simulink model "HoodReleaseModel"  (R2020b)
settings: Solver=VariableStepAuto  StartTime=0.0  StopTime=inf  RelTol=1e-3
libraries: simulink x2
settings Model: Creator=99003785  LastModifiedBy=99003785

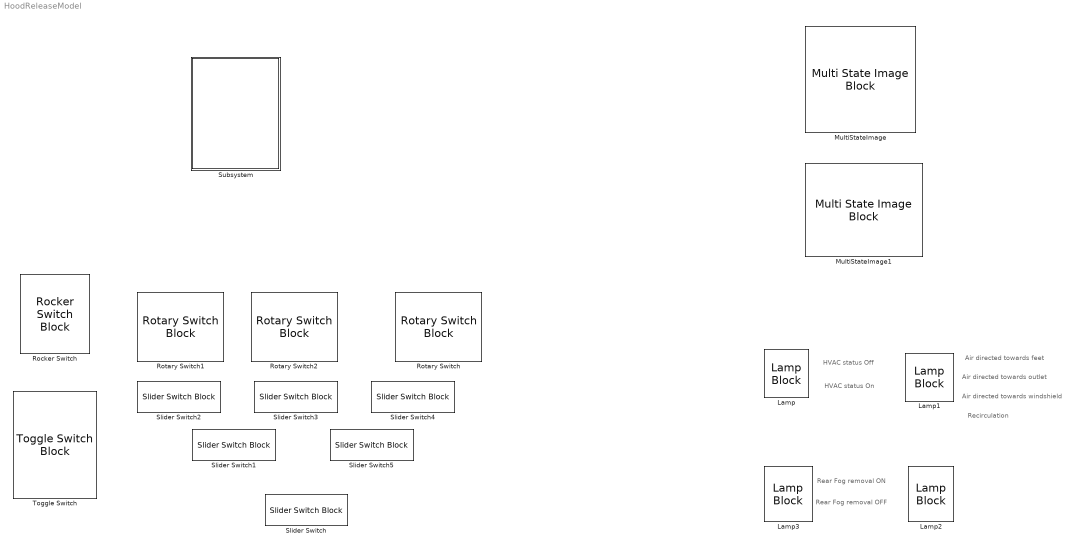
== system HoodReleaseModel ==
  note: Rear Fog removal OFF
  note: Rear Fog removal ON
  note: Recirculation
  note: Air directed towards windshield
  note: Air directed towards outlet
  note: Air directed towards feet
  note: HVAC status Off
  note: HVAC status On
  Lamp{,1..3} (4 alike) : LampBlock
  MultiStateImage : MultiStateImageBlock
  MultiStateImage1 : MultiStateImageBlock
  Rocker Switch : RockerSwitchBlock
      settings: Values={{'On', 'Off'}, [1 0]}
  Rotary Switch : RotarySwitchBlock
      settings: Values={{'Off', 'Low', 'Medium', 'High'}, [0 1 2 3]}
  Rotary Switch1 : RotarySwitchBlock
      settings: Values={{'Off', 'Low', 'Medium', 'High'}, [0 1 2 3]}
  Rotary Switch2 : RotarySwitchBlock
      settings: Values={{'Off', 'AC', 'Heater', 'Air-Vent'}, [0 1 2 3]}
  Slider Switch{,1..5} (6 alike) : SliderSwitchBlock
      settings: Values={{'Off', 'On'}, [0 1]}
  Subsystem : Subsystem
  Toggle Switch : ToggleSwitchBlock
      settings: Values={{'Off', 'On'}, [0 1]}

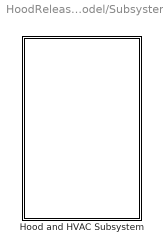
== system HoodReleaseModel/Subsystem ==
  Hood and HVAC Subsystem : Subsystem  TreatAsAtomicUnit=on

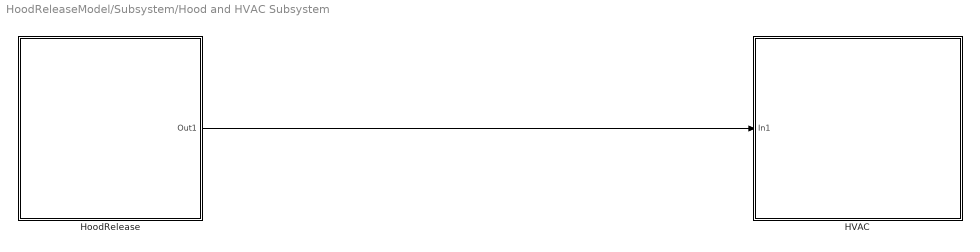
== system HoodReleaseModel/Subsystem/Hood and HVAC Subsystem ==
  HVAC : Subsystem
  HoodRelease : Subsystem
  wires:
  HoodRelease/1(Out1) -> HVAC/1(In1)

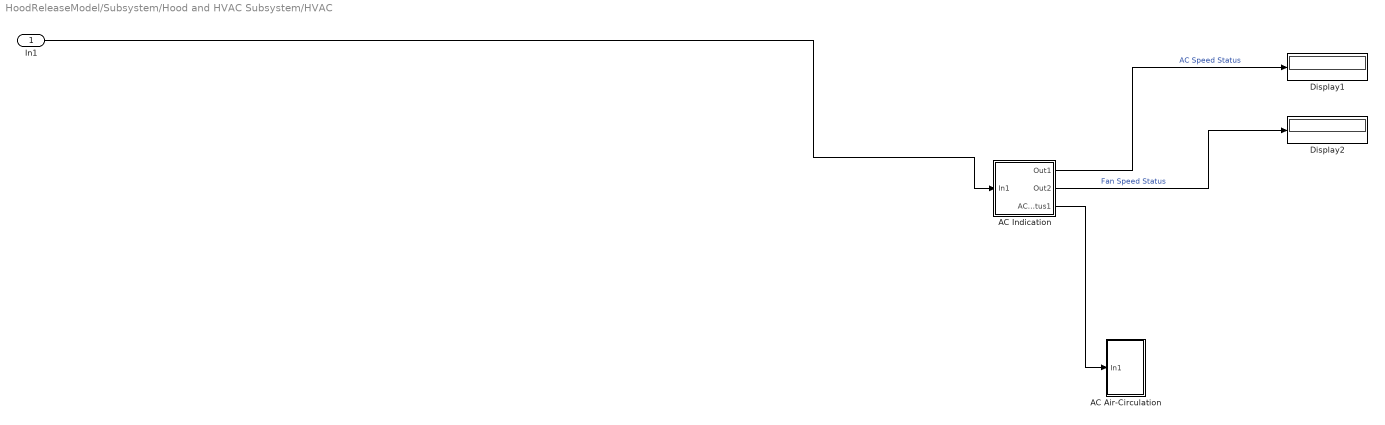
== system HoodReleaseModel/Subsystem/Hood and HVAC Subsystem/HVAC ==
  In1 : Inport
  AC Air-Circulation : Subsystem
  AC Indication : Subsystem
  Display1 : Display
  Display2 : Display
  wires:
  In1/1 -> AC Indication/1(In1)
  AC Indication/1(Out1) -> Display1/1  "AC Speed Status"
  AC Indication/2(Out2) -> Display2/1  "Fan Speed Status"
  AC Indication/3(AC Status1) -> AC Air-Circulation/1(In1)

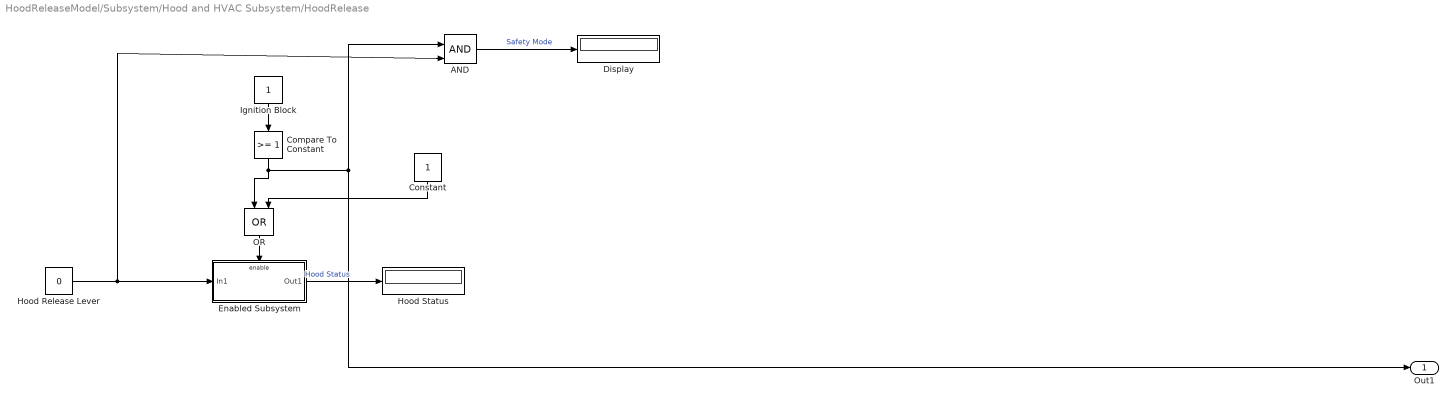
== system HoodReleaseModel/Subsystem/Hood and HVAC Subsystem/HoodRelease ==
  AND : Logic  IconShape=distinctive  AllPortsSameDT=off  OutDataTypeStr=boolean
  Compare To Constant : simulink/Logic and Bit Operations/Compare To Constant  relop=>=  const=1  OutDataTypeStr=boolean
  Constant : Constant
  Display : Display
  Enabled Subsystem : Subsystem  TreatAsAtomicUnit=on
  Hood Release Lever : Constant  Value=0
  Hood Status : Display
  Ignition Block : Constant
  OR : Logic  Operator=OR  IconShape=distinctive  AllPortsSameDT=off  OutDataTypeStr=boolean
  Out1 : Outport
  wires:
  Hood Release Lever/1 -> AND/2, Enabled Subsystem/1(In1)
  Enabled Subsystem/1(Out1) -> Hood Status/1  "Hood Status"
  Constant/1 -> OR/2
  OR/1 -> Enabled Subsystem/Enable
  AND/1 -> Display/1  "Safety Mode"
  Ignition Block/1 -> Compare To Constant/1
  Compare To Constant/1 -> Out1/1, AND/1, OR/1

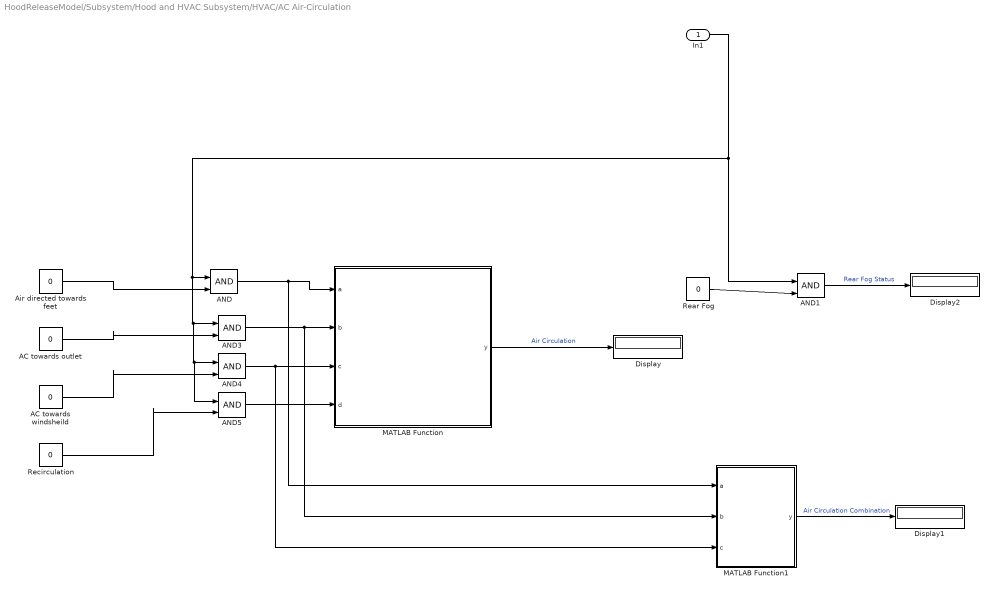
== system HoodReleaseModel/Subsystem/Hood and HVAC Subsystem/HVAC/AC Air-Circulation ==
  In1 : Inport
  AC towards outlet : Constant  Value=0
  AC towards windsheild : Constant  Value=0
  AND{,1,3..5} (5 alike) : Logic  IconShape=distinctive  AllPortsSameDT=off  OutDataTypeStr=boolean
  Air directed towards feet : Constant  Value=0
  Display : Display
  Display1 : Display
  Display2 : Display
  MATLAB Function : MATLAB Function  TreatAsAtomicUnit=on
  MATLAB Function1 : MATLAB Function  TreatAsAtomicUnit=on
  Rear Fog : Constant  Value=0
  Recirculation : Constant  Value=0
  wires:
  AC towards outlet/1 -> AND3/2
  In1/1 -> AND1/1, AND5/1, AND4/1, AND3/1, AND/1
  AND4/1 -> MATLAB Function1/3(c), MATLAB Function/3(c)
  MATLAB Function/1(y) -> Display/1  "Air Circulation"
  Recirculation/1 -> AND5/2
  AC towards windsheild/1 -> AND4/2
  AND/1 -> MATLAB Function1/1(a), MATLAB Function/1(a)
  AND3/1 -> MATLAB Function1/2(b), MATLAB Function/2(b)
  AND5/1 -> MATLAB Function/4(d)
  Air directed towards feet/1 -> AND/2
  MATLAB Function1/1(y) -> Display1/1  "Air Circulation Combination"
  Rear Fog/1 -> AND1/2
  AND1/1 -> Display2/1  "Rear Fog Status"

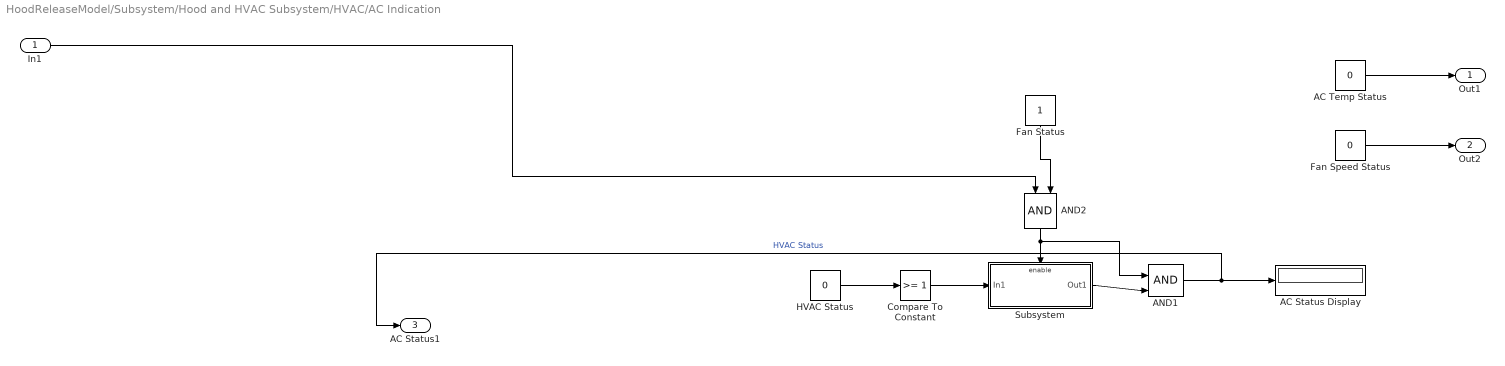
== system HoodReleaseModel/Subsystem/Hood and HVAC Subsystem/HVAC/AC Indication ==
  In1 : Inport
  AC Status Display : Display
  AC Temp Status : Constant  Value=0
  AND1 : Logic  IconShape=distinctive  AllPortsSameDT=off  OutDataTypeStr=boolean
  AND2 : Logic  IconShape=distinctive  AllPortsSameDT=off  OutDataTypeStr=boolean
  Compare To Constant : simulink/Logic and Bit Operations/Compare To Constant  relop=>=  const=1  OutDataTypeStr=boolean
  Fan Speed Status : Constant  Value=0
  Fan Status : Constant
  HVAC Status : Constant  Value=0
  Subsystem : Subsystem
  Out1 : Outport
  Out2 : Outport  Port=2
  AC Status1 : Outport  Port=3
  wires:
  Fan Status/1 -> AND2/2
  In1/1 -> AND2/1
  Fan Speed Status/1 -> Out2/1
  AND2/1 -> AND1/1, Subsystem/Enable
  Subsystem/1(Out1) -> AND1/2
  AND1/1 -> AC Status1/1, AC Status Display/1  "HVAC Status"
  AC Temp Status/1 -> Out1/1
  HVAC Status/1 -> Compare To Constant/1
  Compare To Constant/1 -> Subsystem/1(In1)

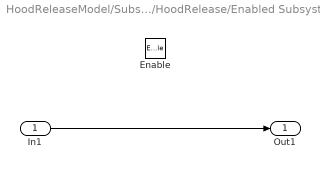
== system HoodReleaseModel/Subsystem/Hood and HVAC Subsystem/HoodRelease/Enabled Subsystem ==
  In1 : Inport
  Enable : EnablePort
  Out1 : Outport  InitialOutput=0  VectorParamsAs1DForOutWhenUnconnected=off
  wires:
  In1/1 -> Out1/1

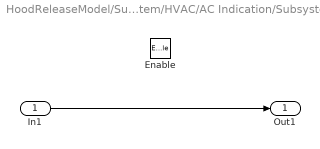
== system HoodReleaseModel/Subsystem/Hood and HVAC Subsystem/HVAC/AC Indication/Subsystem ==
  In1 : Inport
  Enable : EnablePort
  Out1 : Outport
  wires:
  In1/1 -> Out1/1

== matlab function HoodReleaseModel/Subsystem/Hood and HVAC Subsystem/HVAC/AC Air-Circulation/MATLAB Function1 ==
  data: a input; b input; c input; y output
function y = fcn(a,b,c)
    if a==1&& b==1 && c==1
        y=1;
    elseif a==1 && b==1 && c==0
        y=2;
    elseif a==1 && b==0 && c==1
        y=3;
    elseif a==0 && b==1 && c==1
        y=4;
    else
        y=0;
    end

end

== matlab function HoodReleaseModel/Subsystem/Hood and HVAC Subsystem/HVAC/AC Air-Circulation/MATLAB Function ==
  data: a input; b input; y output; c input; d input
function y = fcn(a, b, c, d)
    if a==1 && b==0 && c==0 && d==0
        y=1;
    elseif a==0 && b==1 &&c==0 && d==0
        y=2;
    elseif a==0 && b==0 &&c==1 && d==0
        y=3;
    elseif a==0 && b==0 &&c==0 && d==1
        y=4;
    else
        y=0;
    end
    

end
